simulink model "AdaptiveThreshold"  (R2020a)
settings: Solver=VariableStepAuto  StartTime=0.0  StopTime=10  RelTol=1e-3
libraries: sdolib x1, dspswit3 x1, dspfdesign x1, dspstat3 x1, simulink x1
settings Model: Creator=sbuccelli  LastModifiedBy=diflo

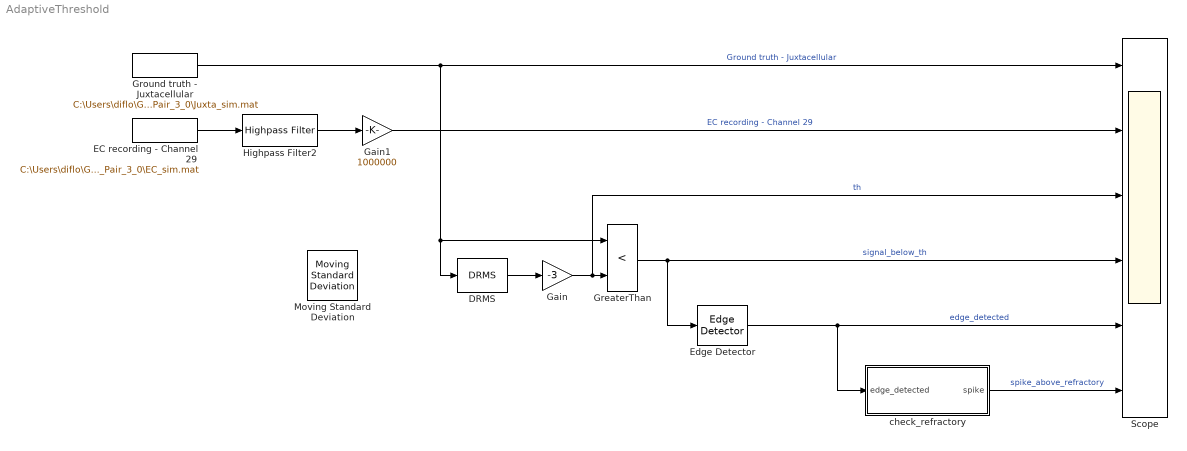
== system AdaptiveThreshold ==
  DRMS : sdolib/RMS Blocks/DRMS  Ts=1/30000
      settings: SourceProductBaseCode=SO
  EC recording - Channel 29 : FromFile  FileName=C:\Users\diflo\Google Drive\IIT - Neuroengineering\Project\WP1\Data\KampffLab\2014_11_25_Pair_3_0\EC_sim.mat  SampleTime=1/30000
  Edge Detector : dspswit3/Edge Detector  InputProcessing=Columns as channels (frame based)
      settings: SourceProductBaseCode=DS
  Gain : Gain  Gain=-3
  Gain1 : Gain  Gain=1000000
  GreaterThan : RelationalOperator  Operator=<  OutDataTypeStr=boolean  RndMeth=Simplest
  Ground truth - Juxtacellular : FromFile  FileName=C:\Users\diflo\Google Drive\IIT - Neuroengineering\Project\WP1\Data\KampffLab\2014_11_25_Pair_3_0\Juxta_sim.mat  SampleTime=1/30000
  Highpass Filter2 : dspfdesign/Highpass Filter  FilterType=IIR  DesignForMinimumOrder=off  FilterOrder=3  StopbandFrequency=1  PassbandFrequency=300  StopbandAttenuation=80  PassbandRipple=0.1  InheritSampleRate=off  SampleRate=30000  SimulateUsing=Interpreted execution  roundingMode=Floor  coeffsDataTypeStr=fixdt(1,16)
  Moving Standard Deviation : dspstat3/Moving Standard Deviation  Method=Sliding window  ForgettingFactorPort=off  SpecifyWindowLength=on  WindowLength=3200  ForgettingFactor=0.9  SimulateUsing=Code generation
      settings: SourceProductBaseCode=DS
  Scope : Scope  NumInputPorts=6
  check_refractory : Subsystem
  wires:
  Ground truth - Juxtacellular/1 -> Scope/1, DRMS/1, GreaterThan/1  "Ground truth - Juxtacellular"
  EC recording - Channel 29/1 -> Highpass Filter2/1
  Edge Detector/1 -> Scope/5, check_refractory/1(edge_detected)  "edge_detected"
  check_refractory/1(spike) -> Scope/6  "spike_above_refractory"
  GreaterThan/1 -> Scope/4, Edge Detector/1  "signal_below_th"
  Gain/1 -> Scope/3, GreaterThan/2  "th"
  DRMS/1 -> Gain/1
  Gain1/1 -> Scope/2  "EC recording - Channel 29"
  Highpass Filter2/1 -> Gain1/1

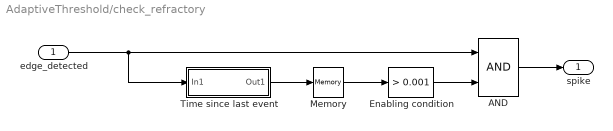
== system AdaptiveThreshold/check_refractory ==
  edge_detected : Inport
  AND : Logic  IconShape=distinctive  AllPortsSameDT=off  OutDataTypeStr=boolean
  Enabling condition : simulink/Logic and Bit Operations/Compare To Constant  relop=>  const=0.001  OutDataTypeStr=boolean
  Memory : Memory  InheritSampleTime=on
  "Time since last event " : Subsystem
  spike : Outport
  wires:
  edge_detected/1 -> "Time since last event "/1(In1), AND/1
  Enabling condition/1 -> AND/2
  Memory/1 -> Enabling condition/1
  "Time since last event "/1(Out1) -> Memory/1
  AND/1 -> spike/1

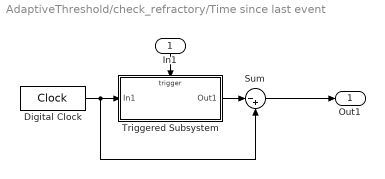
== system AdaptiveThreshold/check_refractory/Time since last event  ==
  In1 : Inport
  Digital Clock : DigitalClock  SampleTime=1/32e3
  Sum : Sum  Inputs=|-+
  Triggered Subsystem : Subsystem  TreatAsAtomicUnit=on
  Out1 : Outport
  wires:
  Digital Clock/1 -> Sum/2, Triggered Subsystem/1(In1)
  Triggered Subsystem/1(Out1) -> Sum/1
  In1/1 -> Triggered Subsystem/Trigger
  Sum/1 -> Out1/1

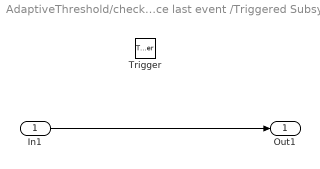
== system AdaptiveThreshold/check_refractory/Time since last event /Triggered Subsystem ==
  In1 : Inport
  Trigger : TriggerPort  VariantControl=Variant
  Out1 : Outport
  wires:
  In1/1 -> Out1/1
